simulink model "LiDAR"  (R2015a)
settings: Solver=ode45  SolverMode=SingleTasking  StartTime=0.0  StopTime=1  FixedStep=0.05  RelTol=1e-3
libraries: simulink x2, simulink_extras x1
settings Model: Creator=Luke  LastModifiedBy=Luke
settings DataIOCC: SignalLoggingSaveFormat=ModelDataLogs
settings OptimizationCC: BlockReduction=off  BooleanDataType=off  ExpressionDepthLimit=2147483647
settings DebuggingCC: SaveWithParameterizedLinksMsg=none  UnderspecifiedInitializationDetection=Classic  MergeDetectMultiDrivingBlocksExec=none  SignalResolutionControl=TryResolveAllWithWarning  MultiTaskDSMMsg=warning  MultiTaskCondExecSysMsg=none  FcnCallInpInsideContextMsg=EnableAllAsWarning  StateNameClashWarn=warning
settings HardwareCC: TargetUnknown=on

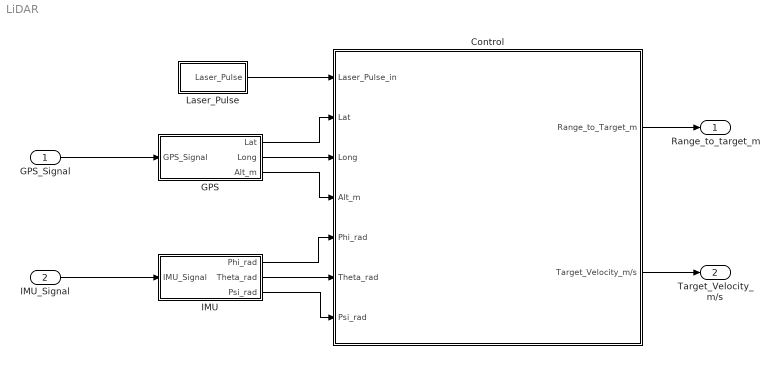
== system LiDAR ==
  GPS_Signal : Inport
  IMU_Signal : Inport  Port=2
  Control : Subsystem
  GPS : Subsystem
  IMU : Subsystem
  Laser_Pulse : Subsystem
  Range_to_target_m : Outport
  Target_Velocity_m/s : Outport  Port=2
  wires:
  GPS/1(Lat) -> Control/2(Lat)
  GPS/2(Long) -> Control/3(Long)
  GPS/3(Alt_m) -> Control/4(Alt_m)
  IMU/2(Theta_rad) -> Control/6(Theta_rad)
  IMU/1(Phi_rad) -> Control/5(Phi_rad)
  IMU/3(Psi_rad) -> Control/7(Psi_rad)
  Laser_Pulse/1(Laser_Pulse) -> Control/1(Laser_Pulse_in)
  GPS_Signal/1 -> GPS/1(GPS_Signal)
  IMU_Signal/1 -> IMU/1(IMU_Signal)
  Control/1(Range_to_Target_m) -> Range_to_target_m/1
  Control/2(Target_Velocity_m/s) -> Target_Velocity_m/s/1

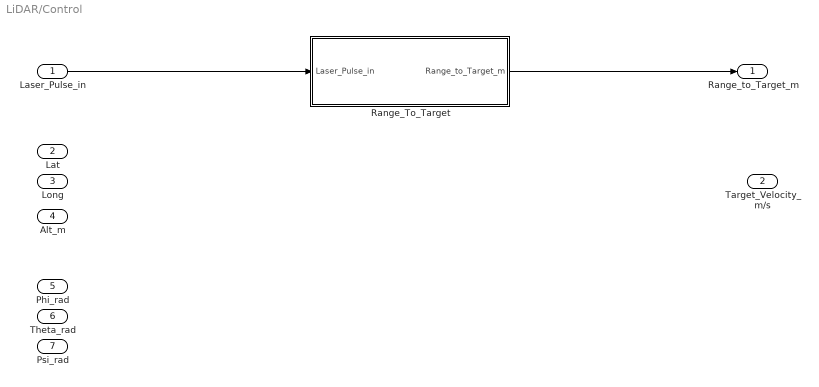
== system LiDAR/Control ==
  Laser_Pulse_in : Inport
  Lat : Inport  Port=2
  Long : Inport  Port=3
  Alt_m : Inport  Port=4
  Phi_rad : Inport  Port=5
  Theta_rad : Inport  Port=6
  Psi_rad : Inport  Port=7
  Range_To_Target : Subsystem
  Range_to_Target_m : Outport
  Target_Velocity_m/s : Outport  Port=2
  wires:
  Range_To_Target/1(Range_to_Target_m) -> Range_to_Target_m/1
  Laser_Pulse_in/1 -> Range_To_Target/1(Laser_Pulse_in)

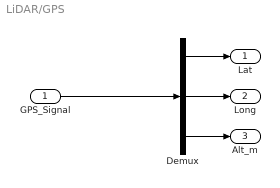
== system LiDAR/GPS ==
  GPS_Signal : Inport
  Demux : Demux  Outputs=3
  Lat : Outport
  Long : Outport  Port=2
  Alt_m : Outport  Port=3
  wires:
  Demux/1 -> Lat/1
  Demux/2 -> Long/1
  Demux/3 -> Alt_m/1
  GPS_Signal/1 -> Demux/1

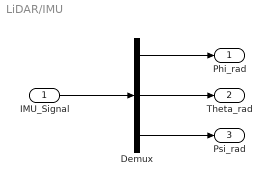
== system LiDAR/IMU ==
  IMU_Signal : Inport
  Demux : Demux  Outputs=3
  Phi_rad : Outport
  Theta_rad : Outport  Port=2
  Psi_rad : Outport  Port=3
  wires:
  Demux/1 -> Phi_rad/1
  Demux/2 -> Theta_rad/1
  Demux/3 -> Psi_rad/1
  IMU_Signal/1 -> Demux/1

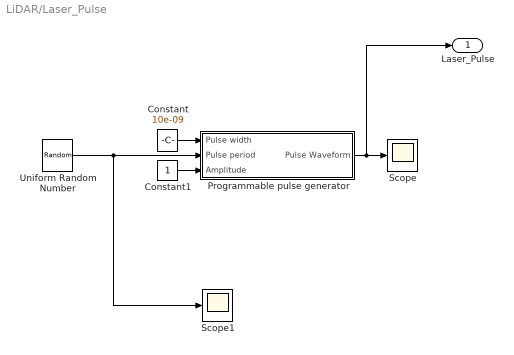
== system LiDAR/Laser_Pulse ==
  Constant : Constant  Value=10e-09
  Constant1 : Constant
  Programmable pulse generator : Subsystem
  Scope : Scope
      settings: YMin=-0  YMax=2  SaveName=ScopeData3
  Scope1 : Scope
      settings: SaveName=ScopeData4
  Uniform Random Number : UniformRandomNumber  Minimum=0  Maximum=0.1  SampleTime=0.01
  Laser_Pulse : Outport
  wires:
  Constant/1 -> Programmable pulse generator/1(Pulse width)
  Constant1/1 -> Programmable pulse generator/3(Amplitude)
  Uniform Random Number/1 -> Programmable pulse generator/2(Pulse period), Scope1/1
  Programmable pulse generator/1(Pulse Waveform) -> Laser_Pulse/1, Scope/1

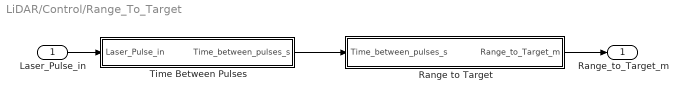
== system LiDAR/Control/Range_To_Target ==
  Laser_Pulse_in : Inport
  Range to Target : Subsystem
  Time Between Pulses : Subsystem
  Range_to_Target_m : Outport
  wires:
  Laser_Pulse_in/1 -> Time Between Pulses/1(Laser_Pulse_in)
  Time Between Pulses/1(Time_between_pulses_s) -> Range to Target/1(Time_between_pulses_s)
  Range to Target/1(Range_to_Target_m) -> Range_to_Target_m/1

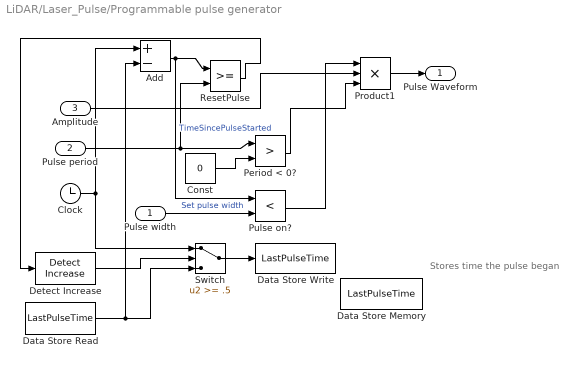
== system LiDAR/Laser_Pulse/Programmable pulse generator ==
  note: Stores time the pulse began
  Pulse width : Inport
  Pulse period : Inport  Port=2
  Amplitude : Inport  Port=3
  Add : Sum  Inputs=+-
  Clock : Clock
  Const : Constant  Value=0
  Data Store Memory : DataStoreMemory  DataStoreName=LastPulseTime
  Data Store Read : DataStoreRead  DataStoreName=LastPulseTime  SampleTime=0
  Data Store Write : DataStoreWrite  DataStoreName=LastPulseTime
  Detect Increase : simulink/Logic and Bit Operations/Detect Increase  vinit=0.0  InputProcessing=Inherited  OutDataTypeStr=uint8
  Period < 0? : RelationalOperator  Operator=>  OutDataTypeStr=boolean
  Product1 : Product  Inputs=3  RndMeth=Zero
  Pulse on? : RelationalOperator  Operator=<  OutDataTypeStr=boolean
  ResetPulse : RelationalOperator  OutDataTypeStr=boolean
  Switch : Switch  Threshold=.5
  Pulse Waveform : Outport
  wires:
  Pulse period/1 -> Period < 0?/1, ResetPulse/2
  Clock/1 -> Add/1, Switch/1
  ResetPulse/1 -> Detect Increase/1
  Product1/1 -> Pulse Waveform/1
  Amplitude/1 -> Product1/2
  Period < 0?/1 -> Product1/3
  Const/1 -> Period < 0?/2
  Switch/1 -> Data Store Write/1
  Data Store Read/1 -> Add/2, Switch/3
  Detect Increase/1 -> Switch/2
  Add/1 -> ResetPulse/1, Pulse on?/1  "TimeSincePulseStarted"
  Pulse on?/1 -> Product1/1
  Pulse width/1 -> Pulse on?/2  "Set pulse width"

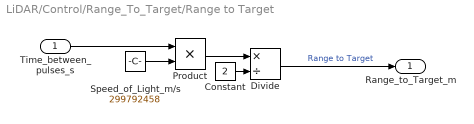
== system LiDAR/Control/Range_To_Target/Range to Target ==
  Time_between_pulses_s : Inport
  Constant : Constant  Value=2
  Divide : Product  Inputs=*/
  Product : Product  RndMeth=Zero
  Speed_of_Light_m/s : Constant  Value=299792458
  Range_to_Target_m : Outport
  wires:
  Speed_of_Light_m/s/1 -> Product/2
  Product/1 -> Divide/1
  Divide/1 -> Range_to_Target_m/1  "Range to Target"
  Constant/1 -> Divide/2
  Time_between_pulses_s/1 -> Product/1

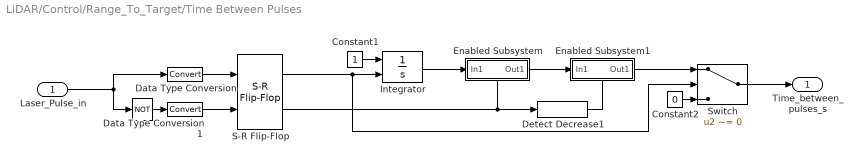
== system LiDAR/Control/Range_To_Target/Time Between Pulses ==
  Laser_Pulse_in : Inport
  " " : Logic  Operator=NOT  AllPortsSameDT=off  OutDataTypeStr=boolean
  Constant1 : Constant
  Constant2 : Constant  Value=0
  Data Type Conversion : DataTypeConversion
  Data Type Conversion1 : DataTypeConversion
  Detect Decrease1 : simulink/Logic and Bit Operations/Detect Decrease  vinit=0.0  InputProcessing=Inherited  OutDataTypeStr=boolean
  Enabled Subsystem : Subsystem  TreatAsAtomicUnit=on
  Enabled Subsystem1 : Subsystem  TreatAsAtomicUnit=on
  Integrator : Integrator  ExternalReset=rising
  S-R Flip-Flop : simulink_extras/Flip Flops/S-R Flip-Flop  initial_condition=0
  Switch : Switch  Criteria=u2 ~= 0
  Time_between_pulses_s : Outport
  wires:
  S-R Flip-Flop/1 -> Switch/2, Integrator/2
  Constant1/1 -> Integrator/1
  Enabled Subsystem/1(Out1) -> Enabled Subsystem1/1(In1)
  " "/1 -> Data Type Conversion1/1
  Data Type Conversion1/1 -> S-R Flip-Flop/2
  Laser_Pulse_in/1 -> " "/1, Data Type Conversion/1
  Data Type Conversion/1 -> S-R Flip-Flop/1
  Integrator/1 -> Enabled Subsystem/1(In1)
  S-R Flip-Flop/2 -> Detect Decrease1/1, Enabled Subsystem/Enable
  Switch/1 -> Time_between_pulses_s/1
  Enabled Subsystem1/1(Out1) -> Switch/1
  Constant2/1 -> Switch/3
  Detect Decrease1/1 -> Enabled Subsystem1/Enable

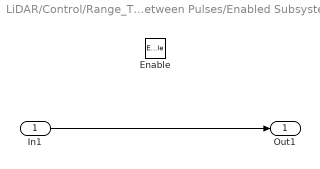
== system LiDAR/Control/Range_To_Target/Time Between Pulses/Enabled Subsystem ==
  In1 : Inport
  Enable : EnablePort
  Out1 : Outport
  wires:
  In1/1 -> Out1/1

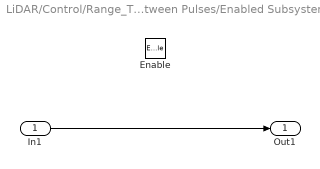
== system LiDAR/Control/Range_To_Target/Time Between Pulses/Enabled Subsystem1 ==
  In1 : Inport
  Enable : EnablePort
  Out1 : Outport
  wires:
  In1/1 -> Out1/1
